simulink model "Sistema"  (R2023a)
settings: Solver=ode15s  StartTime=0.0  StopTime=10  MaxStep=1E-3  RelTol=1e-3
libraries: fl_lib x14, nesl_utility x6, slpidlib x1
settings Model: Creator=lunit  LastModifiedBy=alan_25
settings DataIOCC: SaveFormat=Array  ReturnWorkspaceOutputs=off  TimeSaveName=t
settings DebuggingCC: AlgebraicLoopMsg=none  ArtificialAlgebraicLoopMsg=none  MaxConsecutiveZCsMsg=none  UnconnectedInputMsg=warning  UnconnectedOutputMsg=warning  UnconnectedLineMsg=warning  ModelReferenceExtraNoncontSigs=none  OperatingPointInterfaceChecksumMismatchMsg=none
settings ModelReferenceCC: EnableRefExpFcnMdlSchedulingChecks=on
settings RTWCC: DLArmComputeVersion=19.05

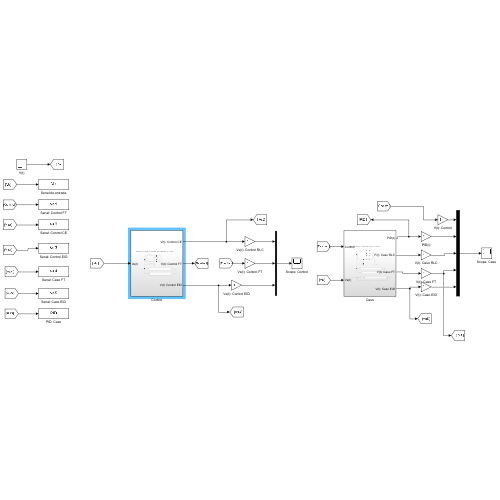
[thumbnail: Simulink's stored preview of the top-level diagram]
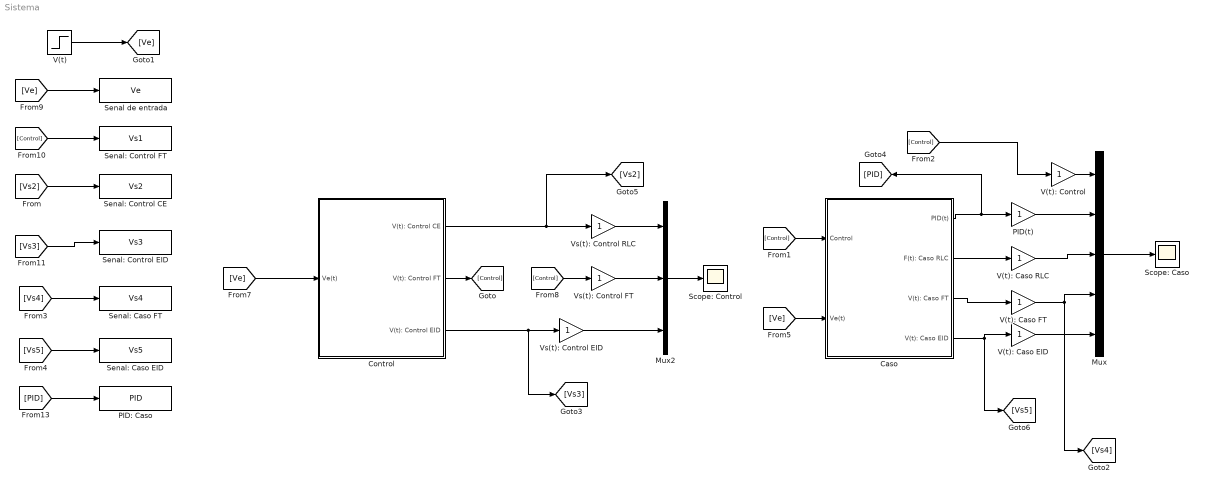
== system Sistema ==
  Caso : Subsystem
  Control : Subsystem
  Mux : Mux  Inputs=5
  Mux2 : Mux  Inputs=3
  PID(t) : Gain
  PID: Caso : ToWorkspace  VariableName=PID  SampleTime=-1
  Scope: Caso : Scope
  Scope: Control : Scope
  Senal de entrada : ToWorkspace  VariableName=Ve  SampleTime=-1
  Senal: Caso EID : ToWorkspace  VariableName=Vs5  SampleTime=-1
  Senal: Caso FT : ToWorkspace  VariableName=Vs4  SampleTime=-1
  Senal: Control CE : ToWorkspace  VariableName=Vs2  SampleTime=-1
  Senal: Control EID : ToWorkspace  VariableName=Vs3  SampleTime=-1
  Senal: Control FT : ToWorkspace  VariableName=Vs1  SampleTime=-1
  V(t) : Step  SampleTime=0
  V(t): Caso EID : Gain
  V(t): Caso FT : Gain
  V(t): Caso RLC : Gain
  V(t): Control : Gain
  Vs(t): Control EID : Gain
  Vs(t): Control FT : Gain
  Vs(t): Control RLC : Gain
  wires:
  [Control] -> Caso/1(Control)
  Control/2(V(t): Control FT) -> [Control]
  [Ve] -> Control/1(Ve(t))
  Mux2/1 -> Scope: Control/1
  Control/1(V(t): Control CE) -> Vs(t): Control RLC/1, [Vs2]
  [Control] -> Vs(t): Control FT/1
  [Ve] -> Senal de entrada/1
  [Control] -> Senal: Control FT/1
  [Vs3] -> Senal: Control EID/1
  [PID] -> PID: Caso/1
  V(t)/1 -> [Ve]
  Vs(t): Control FT/1 -> Mux2/2
  Vs(t): Control RLC/1 -> Mux2/1
  [Control] -> V(t): Control/1
  Caso/1(PID(t)) -> PID(t)/1, [PID]
  PID(t)/1 -> Mux/2
  V(t): Caso RLC/1 -> Mux/3
  V(t): Caso FT/1 -> [Vs4], Mux/4
  [Vs2] -> Senal: Control CE/1
  Caso/2(F(t): Caso RLC) -> V(t): Caso RLC/1
  Caso/3(V(t): Caso FT) -> V(t): Caso FT/1
  [Ve] -> Caso/2(Ve(t))
  Mux/1 -> Scope: Caso/1
  Control/3(V(t): Control EID) -> [Vs3], Vs(t): Control EID/1
  Vs(t): Control EID/1 -> Mux2/3
  [Vs4] -> Senal: Caso FT/1
  Caso/4(V(t): Caso EID) -> [Vs5], V(t): Caso EID/1
  [Vs5] -> Senal: Caso EID/1
  V(t): Control/1 -> Mux/1
  V(t): Caso EID/1 -> Mux/5

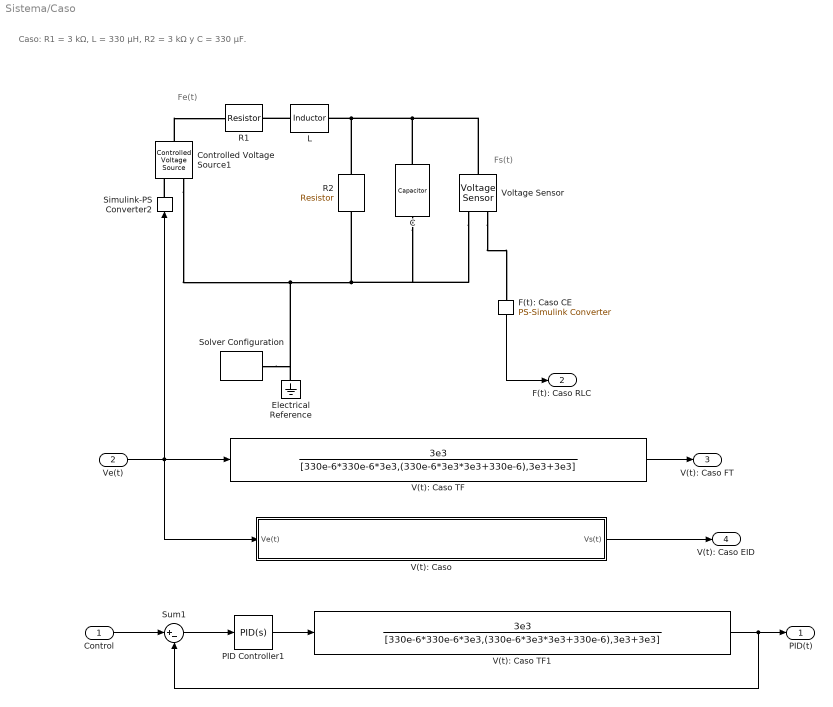
== system Sistema/Caso ==
  note: Caso: R1 = 3 kΩ, L = 330 µH, R2 = 3 kΩ y C = 330 µF.
  note: Fe(t)
  note: Fs(t)
  Control : Inport
  Ve(t) : Inport  Port=2
  C : fl_lib/Electrical/Electrical Elements/Capacitor  c=330 uF  r=1e-6 Ohm  g=0 1/Ohm  i_specify=off  i_priority=None  i=0 A  i_nominal_specify=off  i_nominal_unit=A  i_nominal_value=1  v_specify=off  v_priority=None  v=0 V  v_nominal_specify=off  v_nominal_unit=V  v_nominal_value=1  vc_specify=off  vc_priority=High  vc=0 V  vc_nominal_specify=off  vc_nominal_unit=V  vc_nominal_value=1
  Controlled Voltage Source1 : fl_lib/Electrical/Electrical Sources/Controlled Voltage Source
  Electrical Reference : fl_lib/Electrical/Electrical Elements/Electrical Reference
  F(t): Caso CE : nesl_utility/PS-Simulink Converter  PhysicalDomain=network_engine_domain  SubClassName=ps_output  LeftPortType=input  RightPortType=output  PseudoPeriodic=off  Frequencies=[]  VectorFormat=1-D array  Unit=inherit  AffineConversion=off
  L : fl_lib/Electrical/Electrical Elements/Inductor  l=330 uH  r=0 Ohm  g=1e-9 1/Ohm  i_specify=off  i_priority=None  i=0 A  i_nominal_specify=off  i_nominal_unit=A  i_nominal_value=1  v_specify=off  v_priority=None  v=0 V  v_nominal_specify=off  v_nominal_unit=V  v_nominal_value=1  i_L_specify=off  i_L_priority=High  i_L=0 A  i_L_nominal_specify=off  i_L_nominal_unit=A  i_L_nominal_value=1
  PID Controller1 : slpidlib/PID Controller  Controller=PID  Form=Parallel  TimeDomain=Continuous-time  UseExternalTs=off  SampleTime=-1  IntegratorMethod=Forward Euler  FilterMethod=Forward Euler  ControllerParametersSource=internal  P=128.640661150811  I=3068.81186997597  UseKiTs=off  D=0.100309641900237  N=723.81821555623  UseFilter=on  TunerSelectOption=Transfer Function Based (PID Tuner App)  InitialConditionSource=internal  InitialConditionForIntegrator=0  InitialConditionForFilter=0  DifferentiatorICPrevScaledInput=0  ExternalReset=none  TrackingMode=off  Kt=1  LimitOutput=off  SatLimitsSource=internal  UpperSaturationLimit=inf  LowerSaturationLimit=-inf  LinearizeAsGain=on  AntiWindupMode=none  Kb=1  LimitIntegrator=off  UpperIntegratorSaturationLimit=inf  LowerIntegratorSaturationLimit=-inf  POutMin=[]  POutMax=[]  IOutMin=[]  IOutMax=[]  DOutMin=[]  DOutMax=[]  NOutMin=[]  NOutMax=[]  SumOutMin=[]  SumOutMax=[]  SaturationOutMin=[]  SaturationOutMax=[]  PParamMin=[]  PParamMax=[]  IParamMin=[]  IParamMax=[]  DParamMin=[]  DParamMax=[]  NParamMin=[]  NParamMax=[]  KbParamMin=[]  KbParamMax=[]  KtParamMin=[]  KtParamMax=[]  KbOutMin=[]  KbOutMax=[]  KtOutMin=[]  KtOutMax=[]  IntegratorOutMin=[]  IntegratorOutMax=[]  FilterOutMin=[]  FilterOutMax=[]  SumI1OutMin=[]  SumI1OutMax=[]  SumI2OutMin=[]  SumI2OutMax=[]  SumI3OutMin=[]  SumI3OutMax=[]  SumI4OutMin=[]  SumI4OutMax=[]  SumDOutMin=[]  SumDOutMax=[]  DifferentiatorOutMin=[]  DifferentiatorOutMax=[]  FilterDiffOutCoefMin=[]  FilterDiffOutCoefMax=[]  ReciprocalOutMin=[]  ReciprocalOutMax=[]  SumDenOutMin=[]  SumDenOutMax=[]  SumNumOutMin=[]  SumNumOutMax=[]  DivideOutMin=[]  DivideOutMax=[]  UdiffTsProdOutMin=[]  UdiffTsProdOutMax=[]  NTsProdOutMin=[]  NTsProdOutMax=[]  UintegralTsProdOutMin=[]  UintegralTsProdOutMax=[]  UngainTsProdOutMin=[]  UngainTsProdOutMax=[]  ClampingZeroOutDataTypeStr=Inherit: Inherit via back propagation  ClampingZeroOutMin=[]  ClampingZeroOutMax=[]  FilterDenConstantOutDataTypeStr=Inherit: Inherit via back propagation  FilterDenConstantOutMin=[]  FilterDenConstantOutMax=[]  PCopyOutDataTypeStr=Inherit: Inherit via back propagation  PCopyOutMin=[]  PCopyOutMax=[]  NCopyOutDataTypeStr=Inherit: Inherit via back propagation  NCopyOutMin=[]  NCopyOutMax=[]  IntegratorContinuousStateAttributes=''  IntegratorStateMustResolveToSignalObject=off  IntegratorRTWStateStorageClass=Auto  FilterContinuousStateAttributes=''  FilterStateMustResolveToSignalObject=off  FilterRTWStateStorageClass=Auto  ParallelPVariant=InternalParameters  IdealPVariant=Disabled  IVariant=InternalParameters  DVariant=InternalParameters  IntegratorVariant=Continuous  SatVariant=Disabled  AWVariant=Passthrough  PCopyVariant=Disabled  TRVariant=Disabled  FdbkBlocksVariant=Forward  IdealPFdbkVariant=Disabled  SatFdbkVariant=Disabled  DerivativeFilterVariant=ContFilter  NVariant=InternalParameters  NCopyVariant=Disabled  FilterICVariant=InternalICsFilter  IntegratorICVariant=InternalICs  ExternalResetVariant=Disabled  TRSumVariant=Passthrough  SumFdbkVariant=Disabled  SumVariant=Sum_PID  TsampFilterVariant=InternalTs  TsampNgainVariant=Passthrough  TsampIntegralVariant=Disabled_SignalSpec  ExternalSaturationOutDataTypeStr=Inherit: Same as second input
  R1 : fl_lib/Electrical/Electrical Elements/Resistor  R=3 kOhm  i_specify=off  i_priority=None  i=0 A  i_nominal_specify=off  i_nominal_unit=A  i_nominal_value=1  v_specify=off  v_priority=None  v=0 V  v_nominal_specify=off  v_nominal_unit=V  v_nominal_value=1
  R2 : fl_lib/Electrical/Electrical Elements/Resistor  R=3 kOhm  i_specify=off  i_priority=None  i=0 A  i_nominal_specify=off  i_nominal_unit=A  i_nominal_value=1  v_specify=off  v_priority=None  v=0 V  v_nominal_specify=off  v_nominal_unit=V  v_nominal_value=1
  Simulink-PS Converter2 : nesl_utility/Simulink-PS Converter  PhysicalDomain=network_engine_domain  SubClassName=ps_input  LeftPortType=input  RightPortType=output  PseudoPeriodic=off  Frequencies=[]  NoiseDistribution=none  NoiseParameters=[]  Unit=1  AffineConversion=off  FilteringAndDerivatives=provide  SimscapeFilterOrder=1  InputFilterTimeConstant=0.001  UdotUserProvided=0
  Solver Configuration : nesl_utility/Solver Configuration  PhysicalDomain=network_engine_domain  SubClassName=solver  LeftPortType=input  RightPortType=generic  Tones=[]  Harmonics=[]  SimulateNoise=off  Profile=off  UseLocalSampling=off  EnableSwitchedLinearOptims=on  FrequencyDomain=off  UseCCode=off  RelTol=0.001  AbsTol=1e-06  MinStep=1e-09  ToWorkspace=off  RevertToSquareIcSolve=off  NumHomotopyIterations=100  PhasorMode=off  PhasorModeNumHarmonics=1  ConsistencySolver=NEWTON_FTOL  IndexReductionMethod=DerivativeReplacement  DoDC=off  ResidualTolerance=1e-09  ConsistencyTolSource=GLOBAL  ConsistencyAbsTol=0.001  ConsistencyRelTol=0.001  ConsistencyTolFactor=0.001  UseLocalSolver=off  LocalSolverChoice=NE_BACKWARD_EULER_ADVANCER  ResolveIndetEquations=on  FunctionEvalNumThread=1  LocalSolverSampleTime=0.001  DoFixedCost=off  MaxNonlinIter=3  MaxModeIter=2  ComputeImpulses=off  ImpulseIterations=2  LinearAlgebra=auto  LinearAlgebraNumThread=0  EquationFormulation=NE_TIME_EF  DelaysMemoryBudget=1024  AutomaticFiltering=on  FilteringTimeConstant=0.001  PartitionStorageMethod=AS_NEEDED  PartitionMemoryBudget=1024  PartitionMethod=ROBUST
  Sum1 : Sum  Inputs=|+-
  V(t): Caso : Subsystem
  V(t): Caso TF : TransferFcn  Numerator=[3e3]  Denominator=[330e-6*330e-6*3e3,(330e-6*3e3*3e3+330e-6),3e3+3e3]
  V(t): Caso TF1 : TransferFcn  Numerator=[3e3]  Denominator=[330e-6*330e-6*3e3,(330e-6*3e3*3e3+330e-6),3e3+3e3]
  Voltage Sensor : fl_lib/Electrical/Electrical Sensors/Voltage Sensor
  PID(t) : Outport
  F(t): Caso RLC : Outport  Port=2
  V(t): Caso FT : Outport  Port=3
  V(t): Caso EID : Outport  Port=4
  wires:
  Sum1/1 -> PID Controller1/1
  Control/1 -> Sum1/1
  PID Controller1/1 -> V(t): Caso TF1/1
  V(t): Caso TF/1 -> V(t): Caso FT/1
  F(t): Caso CE/1 -> F(t): Caso RLC/1
  Ve(t)/1 -> V(t): Caso/1(Ve(t)), V(t): Caso TF/1, Simulink-PS Converter2/1
  V(t): Caso/1(Vs(t)) -> V(t): Caso EID/1
  V(t): Caso TF1/1 -> PID(t)/1, Sum1/2
  connections:
  Controlled Voltage Source1/RConn2 -- C/RConn1 -- Voltage Sensor/RConn2 -- R2/RConn1 -- Electrical Reference/LConn1 -- Solver Configuration/RConn1
  L/LConn1 -- R1/RConn1
  Voltage Sensor/LConn1 -- C/LConn1 -- L/RConn1 -- R2/LConn1
  Simulink-PS Converter2/RConn1 -- Controlled Voltage Source1/RConn1
  Voltage Sensor/RConn1 -- F(t): Caso CE/LConn1
  Controlled Voltage Source1/LConn1 -- R1/LConn1

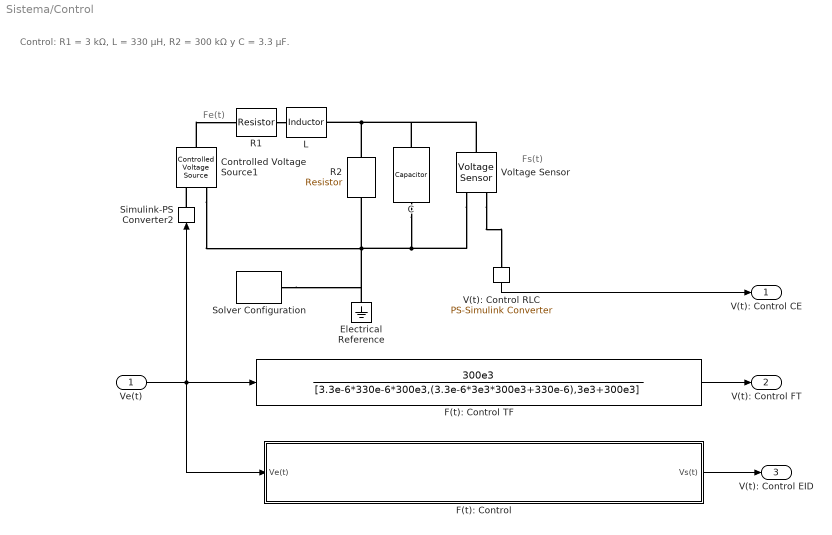
== system Sistema/Control ==
  note: Control: R1 = 3 kΩ, L = 330 µH, R2 = 300 kΩ y C = 3.3 µF.
  note: Fe(t)
  note: Fs(t)
  Ve(t) : Inport
  C : fl_lib/Electrical/Electrical Elements/Capacitor  c=3.3 uF  r=1e-6 Ohm  g=0 1/Ohm  i_specify=off  i_priority=None  i=0 A  i_nominal_specify=off  i_nominal_unit=A  i_nominal_value=1  v_specify=off  v_priority=None  v=0 V  v_nominal_specify=off  v_nominal_unit=V  v_nominal_value=1  vc_specify=off  vc_priority=High  vc=0 V  vc_nominal_specify=off  vc_nominal_unit=V  vc_nominal_value=1
  Controlled Voltage Source1 : fl_lib/Electrical/Electrical Sources/Controlled Voltage Source
  Electrical Reference : fl_lib/Electrical/Electrical Elements/Electrical Reference
  F(t): Control : Subsystem
  F(t): Control TF : TransferFcn  Numerator=[300e3]  Denominator=[3.3e-6*330e-6*300e3,(3.3e-6*3e3*300e3+330e-6),3e3+300e3]
  L : fl_lib/Electrical/Electrical Elements/Inductor  l=330 uH  r=0 Ohm  g=1e-9 1/Ohm  i_specify=off  i_priority=None  i=0 A  i_nominal_specify=off  i_nominal_unit=A  i_nominal_value=1  v_specify=off  v_priority=None  v=0 V  v_nominal_specify=off  v_nominal_unit=V  v_nominal_value=1  i_L_specify=off  i_L_priority=High  i_L=0 A  i_L_nominal_specify=off  i_L_nominal_unit=A  i_L_nominal_value=1
  R1 : fl_lib/Electrical/Electrical Elements/Resistor  R=3 kOhm  i_specify=off  i_priority=None  i=0 A  i_nominal_specify=off  i_nominal_unit=A  i_nominal_value=1  v_specify=off  v_priority=None  v=0 V  v_nominal_specify=off  v_nominal_unit=V  v_nominal_value=1
  R2 : fl_lib/Electrical/Electrical Elements/Resistor  R=300 kOhm  i_specify=off  i_priority=None  i=0 A  i_nominal_specify=off  i_nominal_unit=A  i_nominal_value=1  v_specify=off  v_priority=None  v=0 V  v_nominal_specify=off  v_nominal_unit=V  v_nominal_value=1
  Simulink-PS Converter2 : nesl_utility/Simulink-PS Converter  PhysicalDomain=network_engine_domain  SubClassName=ps_input  LeftPortType=input  RightPortType=output  PseudoPeriodic=off  Frequencies=[]  NoiseDistribution=none  NoiseParameters=[]  Unit=1  AffineConversion=off  FilteringAndDerivatives=provide  SimscapeFilterOrder=1  InputFilterTimeConstant=0.001  UdotUserProvided=0
  Solver Configuration : nesl_utility/Solver Configuration  PhysicalDomain=network_engine_domain  SubClassName=solver  LeftPortType=input  RightPortType=generic  Tones=[]  Harmonics=[]  SimulateNoise=off  Profile=off  UseLocalSampling=off  EnableSwitchedLinearOptims=on  FrequencyDomain=off  UseCCode=off  RelTol=0.001  AbsTol=1e-06  MinStep=1e-09  ToWorkspace=off  RevertToSquareIcSolve=off  NumHomotopyIterations=100  PhasorMode=off  PhasorModeNumHarmonics=1  ConsistencySolver=NEWTON_FTOL  IndexReductionMethod=DerivativeReplacement  DoDC=off  ResidualTolerance=1e-09  ConsistencyTolSource=GLOBAL  ConsistencyAbsTol=0.001  ConsistencyRelTol=0.001  ConsistencyTolFactor=0.001  UseLocalSolver=off  LocalSolverChoice=NE_BACKWARD_EULER_ADVANCER  ResolveIndetEquations=on  FunctionEvalNumThread=1  LocalSolverSampleTime=0.001  DoFixedCost=off  MaxNonlinIter=3  MaxModeIter=2  ComputeImpulses=off  ImpulseIterations=2  LinearAlgebra=auto  LinearAlgebraNumThread=0  EquationFormulation=NE_TIME_EF  DelaysMemoryBudget=1024  AutomaticFiltering=on  FilteringTimeConstant=0.001  PartitionStorageMethod=AS_NEEDED  PartitionMemoryBudget=1024  PartitionMethod=ROBUST
  V(t): Control RLC : nesl_utility/PS-Simulink Converter  PhysicalDomain=network_engine_domain  SubClassName=ps_output  LeftPortType=input  RightPortType=output  PseudoPeriodic=off  Frequencies=[]  VectorFormat=1-D array  Unit=inherit  AffineConversion=off
  Voltage Sensor : fl_lib/Electrical/Electrical Sensors/Voltage Sensor
  V(t): Control CE : Outport
  V(t): Control FT : Outport  Port=2
  V(t): Control EID : Outport  Port=3
  wires:
  Ve(t)/1 -> Simulink-PS Converter2/1, F(t): Control/1(Ve(t)), F(t): Control TF/1
  V(t): Control RLC/1 -> V(t): Control CE/1
  F(t): Control TF/1 -> V(t): Control FT/1
  F(t): Control/1(Vs(t)) -> V(t): Control EID/1
  connections:
  Voltage Sensor/RConn1 -- V(t): Control RLC/LConn1
  Simulink-PS Converter2/RConn1 -- Controlled Voltage Source1/RConn1
  R2/LConn1 -- C/LConn1 -- Voltage Sensor/LConn1 -- L/RConn1
  Voltage Sensor/RConn2 -- Electrical Reference/LConn1 -- Solver Configuration/RConn1 -- R2/RConn1 -- Controlled Voltage Source1/RConn2 -- C/RConn1
  Controlled Voltage Source1/LConn1 -- R1/LConn1
  R1/RConn1 -- L/LConn1

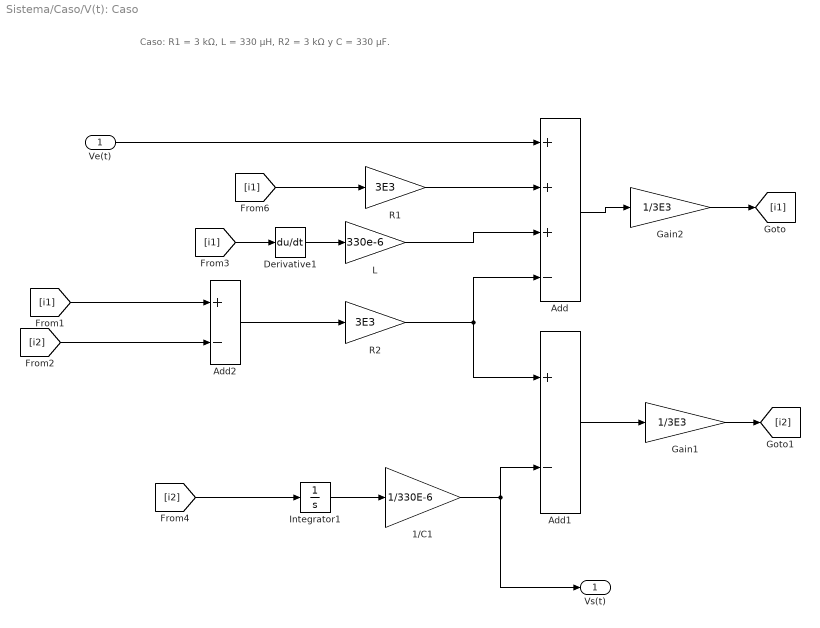
== system Sistema/Caso/V(t): Caso ==
  note: Caso: R1 = 3 kΩ, L = 330 µH, R2 = 3 kΩ y C = 330 µF.
  Ve(t) : Inport
  1/C1 : Gain  Gain=1/330E-6
  Add : Sum  Inputs=+++-
  Add1 : Sum  Inputs=+-
  Add2 : Sum  Inputs=+-
  Derivative1 : Derivative
  Gain1 : Gain  Gain=1/3E3
  Gain2 : Gain  Gain=1/3E3
  Integrator1 : Integrator
  L : Gain  Gain=330e-6
  R1 : Gain  Gain=3E3
  R2 : Gain  Gain=3E3
  Vs(t) : Outport
  wires:
  Add2/1 -> R2/1
  [i2] -> Add2/2
  Ve(t)/1 -> Add/1
  Gain1/1 -> [i2]
  Add/1 -> Gain2/1
  Add1/1 -> Gain1/1
  Gain2/1 -> [i1]
  [i1] -> R1/1
  L/1 -> Add/3
  R2/1 -> Add/4, Add1/1
  1/C1/1 -> Vs(t)/1, Add1/2
  R1/1 -> Add/2
  [i2] -> Integrator1/1
  [i1] -> Add2/1
  [i1] -> Derivative1/1
  Integrator1/1 -> 1/C1/1
  Derivative1/1 -> L/1

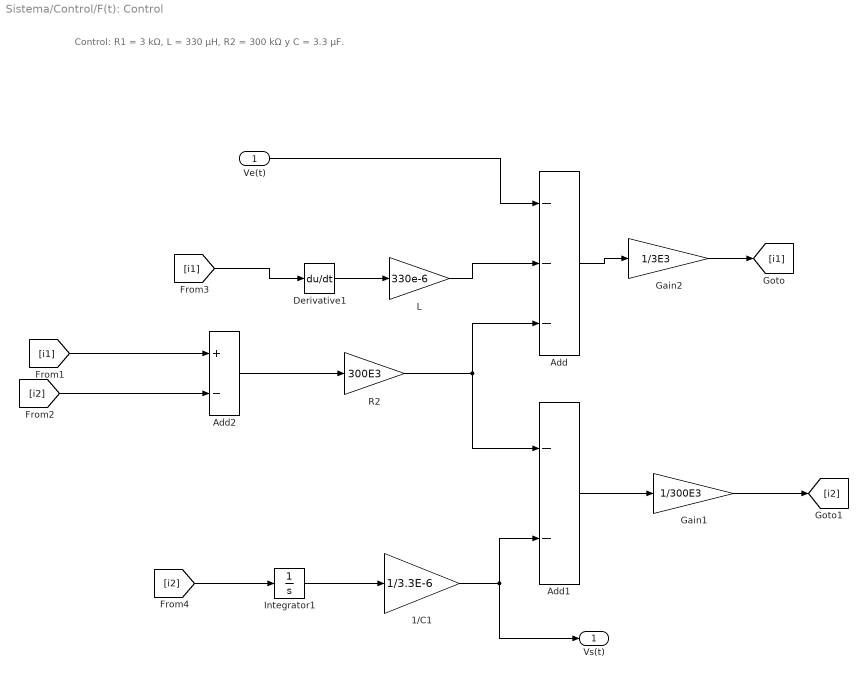
== system Sistema/Control/F(t): Control ==
  note: Control: R1 = 3 kΩ, L = 330 µH, R2 = 300 kΩ y C = 3.3 µF.
  Ve(t) : Inport
  1/C1 : Gain  Gain=1/3.3E-6
  Add : Sum  Inputs=---
  Add1 : Sum  Inputs=--
  Add2 : Sum  Inputs=+-
  Derivative1 : Derivative
  Gain1 : Gain  Gain=1/300E3
  Gain2 : Gain  Gain=1/3E3
  Integrator1 : Integrator
  L : Gain  Gain=330e-6
  R2 : Gain  Gain=300E3
  Vs(t) : Outport
  wires:
  Gain2/1 -> [i1]
  Add/1 -> Gain2/1
  Ve(t)/1 -> Add/1
  [i1] -> Add2/1
  [i2] -> Add2/2
  Add1/1 -> Gain1/1
  Gain1/1 -> [i2]
  [i1] -> Derivative1/1
  Derivative1/1 -> L/1
  [i2] -> Integrator1/1
  Integrator1/1 -> 1/C1/1
  R2/1 -> Add1/1, Add/3
  Add2/1 -> R2/1
  1/C1/1 -> Add1/2, Vs(t)/1
  L/1 -> Add/2
